simulink library "lib_compressor"  (Simulink 7.4)
settings: Solver=ode45  StartTime=0.0  StopTime=10.0  RelTol=1e-3
values from neighbouring files (symbols this model uses):
  x_init_lin = [0.899; 1.126; 0.15; 440; 0]    [comp_rig_parallel_linearized.m]
undefined symbols (not defined in the file or in its folder): u_out
settings Model: Creator=chkajon  LastModifiedBy=chkajon

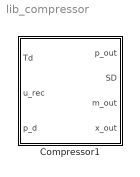
== system lib_compressor ==
  Compressor1 : Subsystem  mask(Compressor){Td_off=0.304, u_in=0.405, u_out=u_out, u_rec=0, t_delay=1, use_dist=off, u_out_dist=0, u_out_time=0}
      mask prompts: Td_off "Torque offset"; u_in "Input valve setting"; u_out "Output valve setting"; u_rec "Recycle valve offset"; t_delay "Recycle valve time delay"; use_dist "Activate output valve disturbance"; u_out_dist "Output valve disturbance magnitudes (up to 2)"; u_out_time "Output valve disturbance times (up to 2)"
      mask help: Compressor with tunable inputs.
      mask init:
      | if use_dist
      |     n = min(length(u_out_dist),length(u_out_time));
      |     if n==0
      |         u_out_dist = [0;0];
      |         u_out_time = [0;0];
      |     elseif n==1
      |         u_out_dist = [u_out_dist(1);0];
      |         u_out_time = [u_out_time(1);0];
      |     else
      |         u_out_dist = [u_out_dist(1);u_out_dist(2)];
      |         u_out_time = [u_out_time(1); u_out_time(2)];
      |     end
      | else
      |     u_out_dist = [0;0];
      |     u_out_time = [0;0];
      | end
      mask TabNameString: Inputs,Inputs,Inputs,Inputs,Inputs,Disturbances,Disturbances,Disturbances

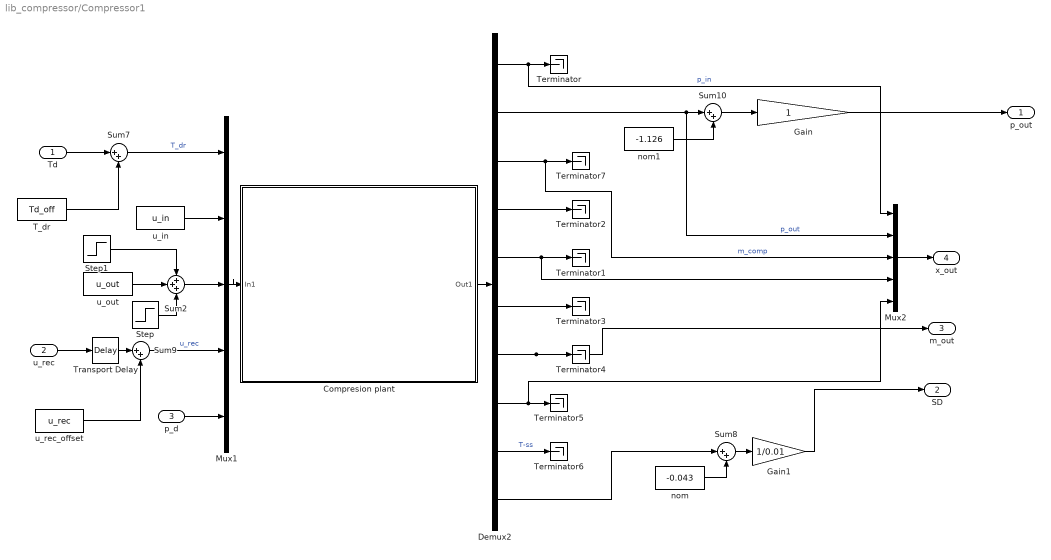
== system lib_compressor/Compressor1 ==
  Td : Inport  OutDataType=fixdt(1, 16)  OutScaling=2^0
  u_rec : Inport  Port=2  OutDataType=fixdt(1, 16)  OutScaling=2^0
  p_d : Inport  Port=3  OutDataType=fixdt(1, 16)  OutScaling=2^0
  Compresion plant : Subsystem
      mask Display: image(imread('comp_plant.jpg'))
  Demux2 : Demux  Outputs=10
  Gain : Gain
  Gain1 : Gain  Gain=1/0.01
  Mux1 : Mux  Inputs=5
  Mux2 : Mux  Inputs=5
  Step : Step  Time=u_out_time(2)  After=u_out_dist(2)  SampleTime=0
  Step1 : Step  Time=u_out_time(1)  After=u_out_dist(1)  SampleTime=0
  Sum{7..10} (4 alike) : Sum  Inputs=|++
  Sum2 : Sum  Inputs=+++
  T_dr : Constant  Value=Td_off
  Terminator{,1..7} (8 alike) : Terminator
  Transport Delay : TransportDelay  DelayTime=t_delay
  nom : Constant  Value=-0.043
  nom1 : Constant  Value=-1.126
  u_in : Constant  Value=u_in
  u_out : Constant  Value=u_out
  u_rec_offset : Constant  Value=u_rec
  p_out : Outport  OutDataType=fixdt(1, 16)  OutScaling=2^0
  SD : Outport  Port=2  OutDataType=fixdt(1, 16)  OutScaling=2^0
  m_out : Outport  Port=3  OutDataType=fixdt(1, 16)  OutScaling=2^0
  x_out : Outport  Port=4  OutDataType=fixdt(1, 16)  OutScaling=2^0
  wires:
  Mux2/1 -> x_out/1
  Demux2/9 -> Terminator6/1  "T-ss"
  Sum2/1 -> Mux1/3
  Step/1 -> Sum2/3
  Transport Delay/1 -> Sum9/1
  p_d/1 -> Mux1/5
  Demux2/10 -> Sum8/1
  Gain1/1 -> SD/1
  Td/1 -> Sum7/1
  u_rec_offset/1 -> Sum9/2
  T_dr/1 -> Sum7/2
  Gain/1 -> p_out/1
  nom1/1 -> Sum10/2
  Sum10/1 -> Gain/1
  Demux2/5 -> Mux2/4, Terminator1/1
  Demux2/1 -> Mux2/1, Terminator/1  "p_in"
  Demux2/2 -> Mux2/2, Sum10/1  "p_out"
  Sum8/1 -> Gain1/1
  nom/1 -> Sum8/2
  Sum9/1 -> Mux1/4  "u_rec"
  Sum7/1 -> Mux1/1  "T_dr"
  u_rec/1 -> Transport Delay/1
  u_out/1 -> Sum2/2
  Demux2/7 -> Terminator4/1, m_out/1
  Demux2/8 -> Mux2/5, Terminator5/1
  Demux2/6 -> Terminator3/1
  u_in/1 -> Mux1/2
  Mux1/1 -> Compresion plant/1(In1)
  Compresion plant/1(Out1) -> Demux2/1
  Step1/1 -> Sum2/1
  Demux2/3 -> Mux2/3, Terminator7/1  "m_comp"
  Demux2/4 -> Terminator2/1

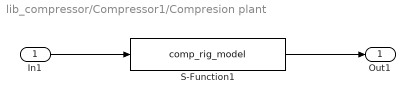
== system lib_compressor/Compressor1/Compresion plant ==
  In1 : Inport
  S-Function1 : S-Function  FunctionName=comp_rig_model  Parameters=[], x_init_lin  EnableBusSupport=off
  Out1 : Outport
  wires:
  In1/1 -> S-Function1/1
  S-Function1/1 -> Out1/1
